simulink model "mpc_model_dual_module"  (R2019a)
settings: Solver=FixedStepAuto  StartTime=0.0  StopTime=Tfinal  RelTol=1e-3
values from neighbouring files (symbols this model uses):
  A = [-0.0285 -0.0014; -0.0371 -0.1476]    [model.m]
  DCLINK_Cap = 1000e-12    (= 1e-09)    [mpc_model_parameters.m]    (also in mpc_model_parameters_dual_module.m = 0.001)
  FluxPM = MeanInducedVoltagePeak/(2*pi*100)    [mpc_model_parameters.m]    (also in mpc_model_parameters_dual_module.m)
  Inertia = 1e-2    (= 0.01)    [mpc_model_parameters.m]    (also in mpc_model_parameters_dual_module.m)
  iqrated = Trated/(1.5*PolePairs*FluxPM)    [mpc_model_parameters.m]    (also in mpc_model_parameters_dual_module.m)
  Ls = 3.5e-3    (= 0.0035)    [MPC_id_iq.m]    (also in mpc_model_parameters.m = 0.00351; mpc_model_parameters_dual_module.m = 0.00351)
  M1_FaultTime = 0.5    [mpc_model_parameters_dual_module.m]
  MeanLd = (1/12)*(Module1Phase_A_Ld+Module1Phase_B_Ld+Module1Phase_C_Ld+     Module2Phase_A_Ld+Module2Phase_B_Ld+Module2Phase_C_Ld+     Module3Phase_A_Ld+Module3Phase_B_Ld+Module3Phase_C_Ld+     Module4Phase_A_Ld+Module4Phase_B_Ld+Module4Phase_C_Ld)    [mpc_model_parameters.m]    (also in mpc_model_parameters_dual_module.m)
  MeanLq = (1/12)*(Module1Phase_A_Lq+Module1Phase_B_Lq+Module1Phase_C_Lq+     Module2Phase_A_Lq+Module2Phase_B_Lq+Module2Phase_C_Lq+     Module3Phase_A_Lq+Module3Phase_B_Lq+Module3Phase_C_Lq+     Module4Phase_A_Lq+Module4Phase_B_Lq+Module4Phase_C_Lq)    [mpc_model_parameters.m]    (also in mpc_model_parameters_dual_module.m)
  PolePairs = 10    [mpc_model_parameters.m]    (also in mpc_model_parameters_dual_module.m)
  Rin = 1e-3    (= 0.001)    [mpc_model_parameters.m]    (also in mpc_model_parameters_dual_module.m)
  Rs = 0.531    [Loss_Distribution.m]    (also in MPC_id_iq.m; mpc_model_parameters.m = 0.321; mpc_model_parameters_dual_module.m = 0.321)
  Sampling_time = 1e-6    (= 1e-06)    [mpc_model_parameters.m]    (also in mpc_model_parameters_dual_module.m)
  SpeedRef1 = 50    [mpc_model_parameters.m]    (also in mpc_model_parameters_dual_module.m = 300)
  SpeedRef2 = 100    [mpc_model_parameters.m]    (also in mpc_model_parameters_dual_module.m = 300)
  SpeedRefUpdateTime = 0.25    [mpc_model_parameters.m]    (also in mpc_model_parameters_dual_module.m = 0.75)
  Tload1 = 5    [mpc_model_parameters.m]    (also in mpc_model_parameters_dual_module.m = 20)
  Tload2 = 10    [mpc_model_parameters.m]    (also in mpc_model_parameters_dual_module.m = 20)
  TloadUpdateTime = 0.5    [mpc_model_parameters.m]    (also in mpc_model_parameters_dual_module.m = 2)
  Vdc = 50    [mpc_model_parameters.m]    (also in mpc_model_parameters_dual_module.m = 270)
  Vin = Vdc + Rin*(Pout/Vdc)    (= 50.04)    [mpc_model_parameters.m]    (also in mpc_model_parameters_dual_module.m = 270.007407407)
  ViscousFriction = 1e-3    (= 0.001)    [mpc_model_parameters.m]    (also in mpc_model_parameters_dual_module.m)
undefined symbols (not defined in the file or in its folder): DiscIntNeverNeededParam
libraries: powerlib x24, dspswit3 x12, fl_lib x5, simulink x3, nesl_utility x3, powerlib_meascontrol x2, sdl_lib x1
(part 2 of 2)

== matlab function mpc_model_dual_module/M2_prediction ==
  data: DutyA output; DutyB output; DutyC output; iqref input; id input; iq input; Ld input; Lq input; Rs input; PolePairs input; wmech input; FluxPM input; Vdc input; ref_frame_position input; switching_pulse input; DutyA_prev input; DutyB_prev input; DutyC_prev input; clock input; vectortableupdatetime input; fsw_out_prev input; fsw_out output; IqRipplePrediction output; IqRipplePredictionPrev input
function [DutyA, DutyB, DutyC, fsw_out, IqRipplePrediction]  = fcn(iqref,id, iq, Ld, Lq, Rs,PolePairs,wmech,FluxPM,Vdc,ref_frame_position,switching_pulse,DutyA_prev, DutyB_prev, DutyC_prev, clock,vectortableupdatetime,fsw_out_prev, IqRipplePredictionPrev)

Ls = Lq;
iN = 11.7362; %this is the rated value of the iq
idref = 0;
cost = zeros(1,8);
ud_1 = zeros(1,8);
uq_1 = zeros(1,8);
% fsw_options = [5000; 10000; 15000; 20000; 25000; 30000; 35000; 40000];
fsw_max = 40000;
fsw_options = 1000:1000:fsw_max;
cost = zeros(1,numel(fsw_options));
ud_1 = zeros(1,numel(fsw_options));
uq_1 = zeros(1,numel(fsw_options));
iqripple = zeros(1,numel(fsw_options));
VoltageDuring_T1 = zeros(1,numel(fsw_options));
VoltageDuring_T2 = zeros(1,numel(fsw_options));
VoltageDuring_T0 = zeros(1,numel(fsw_options));
magnitude_1 = zeros(1,numel(fsw_options));

T1_1 =  zeros(1,numel(fsw_options));
T2_1 =  zeros(1,numel(fsw_options));
T0_1 =  zeros(1,numel(fsw_options));
ma_1 =  zeros(1,numel(fsw_options)); 
Valfa_1 = zeros(1,numel(fsw_options)); 
Vbeta_1 = zeros(1,numel(fsw_options)); 
ma_1 = zeros(1,numel(fsw_options)); 

iq_delta_T1_1 =  zeros(1,numel(fsw_options));
iq_delta_T2_1 =  zeros(1,numel(fsw_options));
iq_delta_T0_1 =  zeros(1,numel(fsw_options));
VoltageVectorAngleAlfa_1 = zeros(1,numel(fsw_options));
VoltageVectorAngle_1 = zeros(1,numel(fsw_options));

if(switching_pulse==1)
    
    for i = 1:numel(fsw_options)
        % calculate vd vq
        ud_1(i) = Rs*id + Ld*fsw_options(i)*(idref-id)-PolePairs*wmech*Lq*iq;
        uq_1(i) = Rs*iq + Lq*fsw_options(i)*(iqref-iq)+PolePairs*wmech*(Ld*id+FluxPM);
        
        magnitude_1(i) = sqrt(ud_1(i)^2+uq_1(i)^2);
        
        Valfa_1(i) = sin(ref_frame_position)*ud_1(i)+cos(ref_frame_position)*uq_1(i);
        Vbeta_1(i) =-cos(ref_frame_position)*ud_1(i)+sin(ref_frame_position)*uq_1(i);     
        
        VoltageVectorAngle_1(i) = atan2(Vbeta_1(i),Valfa_1(i))+4*pi;
        VoltageVectorAngleAlfa_1(i) = mod(VoltageVectorAngle_1(i),pi/3);
        
        ma_1(i) = magnitude_1(i)/(Vdc/sqrt(3));
        
        T1_1(i) = (1/fsw_options(i))*ma_1(i)*sin(pi/3-VoltageVectorAngleAlfa_1(i));
        T2_1(i) = (1/fsw_options(i))*ma_1(i)*sin(VoltageVectorAngleAlfa_1(i));
        T0_1(i) = (1/fsw_options(i))-T1_1(i)-T2_1(i);        
        
        VoltageDuring_T1(i) = 2/3*Vdc-magnitude_1(i);
        VoltageDuring_T2(i) = 2/3*Vdc-magnitude_1(i);
        VoltageDuring_T0(i) = -magnitude_1(i);
        
        iq_delta_T1_1(i) = VoltageDuring_T1(i)*T1_1(i)/Ls;
        iq_delta_T2_1(i) = VoltageDuring_T2(i)*T2_1(i)/Ls;
        iq_delta_T0_1(i) = -VoltageDuring_T0(i)*T0_1(i)/Ls;
        
        iqripple(i) = iq_delta_T1_1(i)+iq_delta_T2_1(i)+iq_delta_T0_1(i);
        
        %predict the future output
        id_1 = id + (1/fsw_options(i))*(ud_1(i)/Ld-Rs/Ld*id+Lq/Ld*PolePairs*wmech*iq);
        iq_1 = iq + (1/fsw_options(i))*(uq_1(i)*Lq-Rs/Lq*iq-Ld/Lq*PolePairs*wmech*id-FluxPM*PolePairs*wmech/Lq);
        Te_1 = 1.5*PolePairs*(FluxPM*iq_1+0*(Ld-Lq)*id_1*iq_1); % reluctance torque component is multiplied by 0, since it caused unreasonable torque values.
        
        %calculate the cost
        if(abs(iq_1)>30)||(abs(Te_1)>50)
            protection = inf;
        else
            protection = 0;
        end
        cost(i) = (iqripple(i)/iN)^2*10000+100000*((iqref-iq_1)/iN)^2+((idref-id_1)/iN)^2*15+protection+fsw_options(i)/fsw_max*50*30;%+IqRipplePredictionPrev^2*100000000;
        
    end
    
    [mincostval, index] = min(cost);
    
    DutyA = 0;
    DutyB = 0;
    DutyC = 0;
    vds_1 = ud_1(index);
    vqs_1 = uq_1(index);
    fsw_out = fsw_options(index);
    
%     Valfa = sin(ref_frame_position)*vds_1+cos(ref_frame_position)*vqs_1;
%     Vbeta =-cos(ref_frame_position)*vds_1+sin(ref_frame_position)*vqs_1;
%     VoltageVectorAngle = atan2(Vbeta,Valfa)+4*pi;
%     VoltageVectorAngleAlfa = mod(VoltageVectorAngle,pi/3);
%     Magnitude =  sqrt(Valfa^2+Vbeta^2);
%     ma = Magnitude/(Vdc/sqrt(3));
    VoltageVectorAngle = VoltageVectorAngle_1(index);
    Tsw = 1/fsw_out;
%     T1 = Tsw*ma*sin(pi/3-VoltageVectorAngleAlfa);
%     T2 = Tsw*ma*sin(VoltageVectorAngleAlfa);
%     T0 = Tsw-T1-T2;
    T1 = T1_1(index);
    T2 = T2_1(index);
    T0 = T0_1(index);
    
%     Vx_in_T0 = -Magnitude;
%     Vx_in_T1 = 2/3*Vdc-Magnitude;
%     Vx_in_T2 = 2/3*Vdc-Magnitude;
%     
%     delta_I_in_T0 = Vx_in_T0*T0/Ls;
%     delta_I_in_T1 = Vx_in_T1*T1/Ls;
%     delta_I_in_T2 = Vx_in_T2*T2/Ls;
    
%     IqRipplePrediction = (delta_I_in_T0+delta_I_in_T1+delta_I_in_T2)/3;
    IqRipplePrediction = iqripple(index);
    if (mod(VoltageVectorAngle, 2*pi)<=pi/3)&&(mod(VoltageVectorAngle, 2*pi)>=0)  % sector 1
        DutyA = (T1+T2+T0/2)/Tsw;
        DutyB = (T2+T0/2)/Tsw;
        DutyC = (T0/2)/Tsw;
        sectornumber = 1;
        return;
    end
    if (mod(VoltageVectorAngle, 2*pi)<=2*pi/3)&&(mod(VoltageVectorAngle, 2*pi)>=pi/3)  % sector 2
        DutyA = (T1+T0/2)/Tsw;
        DutyB = (T1+T2+T0/2)/Tsw;
        DutyC = (T0/2)/Tsw;
        sectornumber = 2;
        return;
    end
    if (mod(VoltageVectorAngle, 2*pi)<=pi)&&(mod(VoltageVectorAngle, 2*pi)>=2*pi/3)  % sector 3
        if(mod(VoltageVectorAngle, pi)==0)
            DutyA = (T0/2)/Tsw;
            DutyB = (T1+T0/2)/Tsw;
            DutyC = (T1+T2+T0/2)/Tsw;
        else
            DutyA = (T0/2)/Tsw;
            DutyB = (T1+T2+T0/2)/Tsw;
            DutyC = (T2+T0/2)/Tsw;
        end
        sectornumber = 3;
        return;
    end
    if (mod(VoltageVectorAngle, 2*pi)<=4*pi/3)&&(mod(VoltageVectorAngle, 2*pi)>=pi)  % sector 4
        DutyA = (T0/2)/Tsw;
        DutyB = (T1+T0/2)/Tsw;
        DutyC = (T1+T2+T0/2)/Tsw;
        sectornumber = 4;
        return;
    end
    if (mod(VoltageVectorAngle, 2*pi)<=5*pi/3)&&(mod(VoltageVectorAngle, 2*pi)>=4*pi/3)  % sector 5
        DutyA = (T2+T0/2)/Tsw;
        DutyB = (T0/2)/Tsw;
        DutyC = (T1+T2+T0/2)/Tsw;
        sectornumber = 5;
        return;
    end
    if (mod(VoltageVectorAngle, 2*pi)<=2*pi)&&(mod(VoltageVectorAngle, 2*pi)>=5*pi/3)  % sector 6
        DutyA = (T1+T2+T0/2)/Tsw;
        DutyB = (T0/2)/Tsw;
        DutyC = (T1+T0/2)/Tsw;
        sectornumber = 6;
        return;
    end
    
else %switching pulse
    
    fsw_out = fsw_out_prev;
    DutyA = DutyA_prev;
    DutyB = DutyB_prev;
    DutyC = DutyC_prev;
    IqRipplePrediction = IqRipplePredictionPrev;
end

== matlab function mpc_model_dual_module/module 1 abc to dq0 ==
  data: ids output; iqs output; ias input; ibs input; ics input; ref_frame_position input; i0 output
function [ids,iqs,i0 ]  = fcn(ias,ibs,ics,ref_frame_position)





ids = 2/3*(ias*sin(ref_frame_position)+ibs*sin(ref_frame_position-2*pi/3)+ics*sin(ref_frame_position+2*pi/3));
iqs =  2/3*(ias*cos(ref_frame_position)+ibs*cos(ref_frame_position-2*pi/3)+ics*cos(ref_frame_position+2*pi/3));
i0 = 2/3*1/2*(ias+ibs+ics);
% iqs = (vqs-fluxlinkage_qs_derivative-ref_frame_velocity*fluxlinkage_ds)/rs;
% ids = (vds-fluxlinkage_ds_derivative+ref_frame_velocity*fluxlinkage_qs)/rs;

== matlab function mpc_model_dual_module/MATLAB Function1 ==
  data: pulse input; inputwave input; outputwave output
function outputwave  = fcn(pulse, inputwave)

persistent state

if isempty(state)
state = 0;
end

if(pulse==1)
    state = state +1;
end

if(mod(state,2)==1)
    outputwave = inputwave;
    return;
end
if(mod(state,2)==0)
    outputwave = 1-inputwave;
    return;
end

outputwave = 5;

== matlab function mpc_model_dual_module/MATLAB Function2 ==
  data: pulse input; inputwave input; outputwave output
function outputwave  = fcn(pulse, inputwave)

persistent state

if isempty(state)
state = 0;
end

if(pulse==1)
    state = state +1;
end

if(mod(state,2)==1)
    outputwave = inputwave;
    return;
end
if(mod(state,2)==0)
    outputwave = 1-inputwave;
    return;
end

outputwave = 5;
